simulink model "Output_Only_Simulation"  (R2018b)
settings: Solver=FixedStepDiscrete  StartTime=0.0  StopTime=inf  FixedStep=0.01  RelTol=1e-3
settings Model: EnablePacing=on  PacingRate=2  Creator=Daniele Nava  LastModifiedBy=Daniele Nava

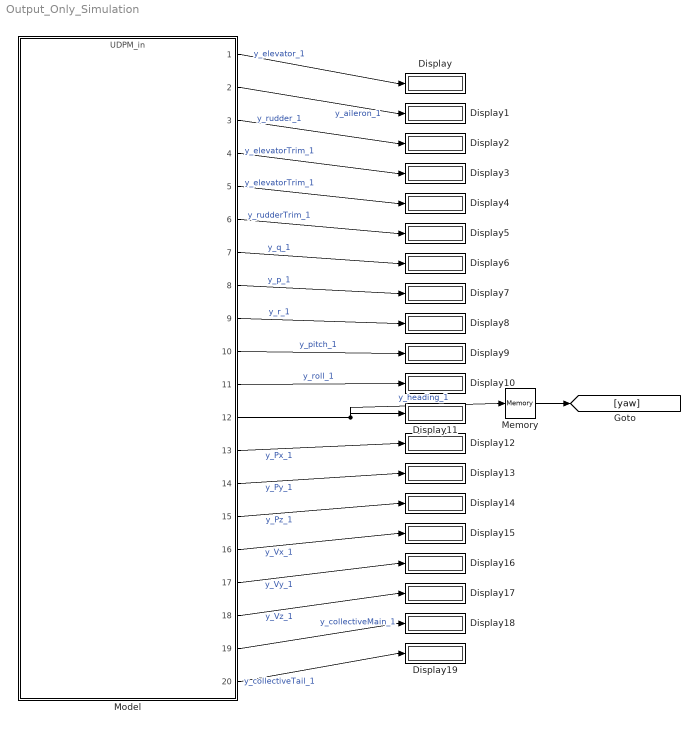
== system Output_Only_Simulation ==
  Display{,1..19} (20 alike) : Display
  Memory : Memory
  Model : ModelReference  ModelNameDialog=UDPM_in.slx  SimulationMode=Normal  ModelReferenceVersion=1.11
  wires:
  Model/2 -> Display1/1  "y_aileron_1"
  Model/9 -> Display8/1  "y_r_1"
  Model/17 -> Display16/1  "y_Vy_1"
  Model/18 -> Display17/1  "y_Vz_1"
  Model/19 -> Display18/1  "y_collectiveMain_1"
  Model/10 -> Display9/1  "y_pitch_1"
  Model/13 -> Display12/1  "y_Px_1"
  Model/14 -> Display13/1  "y_Py_1"
  Model/12 -> Memory/1, Display11/1  "y_heading_1"
  Model/4 -> Display3/1  "y_elevatorTrim_1"
  Model/5 -> Display4/1  "y_elevatorTrim_1"
  Model/20 -> Display19/1  "y_collectiveTail_1"
  Model/8 -> Display7/1  "y_p_1"
  Model/7 -> Display6/1  "y_q_1"
  Model/16 -> Display15/1  "y_Vx_1"
  Model/15 -> Display14/1  "y_Pz_1"
  Model/1 -> Display/1  "y_elevator_1"
  Model/11 -> Display10/1  "y_roll_1"
  Model/3 -> Display2/1  "y_rudder_1"
  Model/6 -> Display5/1  "y_rudderTrim_1"
  Memory/1 -> [yaw]
